simulink model "untitled"  (R2023a)
settings: Solver=VariableStepAuto  StartTime=0.0  StopTime=10.0  RelTol=1e-3
(part 1 of 2)
settings Model: Creator=green  LastModifiedBy=green

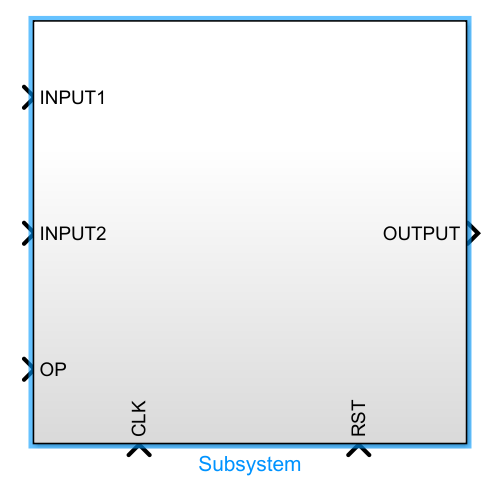
[thumbnail: Simulink's stored preview of the top-level diagram]
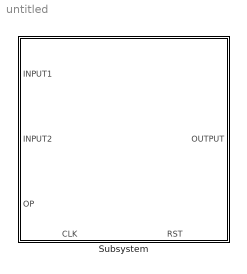
== system untitled ==
  Subsystem : Subsystem
      settings: PortSchema="{\"entries\":[{\"content\":{\"sides\":[{\"content\":{\"connectorIds\":[\"In1\",\"In2\",\"In3\"]},\"type\":\"ConnectorPlacement.EquallySpacedRectSide\",\"uuid\":\"37e95da7-9205-457f-9e39-3ce645baf6b0\"},{\"content\":{\"connectorIds\":[\"Out1\"],\"side\":\"RIGHT\"},\"type\":\"ConnectorPlacement.EquallySpacedRectSide\",\"uuid\":\"fefd857f-f6cb-479d-9e10-fdb7bd1a36ee\"},{\"content\":{\"side\":\"TOP\"},\"type\":\"ConnectorPlacement.EquallySpacedRectSide\",\"uuid\":\"cee60b90-4321-4370-ba97-5c42913d2398\"},{\"content\":{\"connectorIds\":[\"In4\",\"In5\"],\"side\":\"BOTTOM\"},\"type\":\"ConnectorPlacement.EquallySpacedRectSide\",\"uuid\":\"580bfb33-9847-4a2b-9363-58d08870a9b2\"}]},\"type\":\"ConnectorPlacement.EquallySpacedConnector\",\"uuid\":\"096c5676-b756-43ee-88e7-cfe97f701f61\"}],\"packageUris\":[\"http://schema.mathworks.com/mf0/Connector/R2020b\"],\"version\":\"1.0\"}"

== system untitled/Subsystem ==
  INPUT1 : Inport
  INPUT2 : Inport  Port=2
  OP : Inport  Port=3
  CLK : Inport  Port=4
  RST : Inport  Port=5
  AdjustingStage : Subsystem
  ComparingStage : Subsystem
  REG0 : Subsystem
      settings: PortSchema="{\"entries\":[{\"content\":{\"sides\":[{\"content\":{\"connectorIds\":[\"In1\",\"In2\",\"In3\"]},\"type\":\"ConnectorPlacement.EquallySpacedRectSide\",\"uuid\":\"0bf5a9f9-0a2e-40a8-8f36-13e781bf7f7c\"},{\"content\":{\"connectorIds\":[\"Out1\",\"Out2\",\"Out3\"],\"side\":\"RIGHT\"},\"type\":\"ConnectorPlacement.EquallySpacedRectSide\",\"uuid\":\"64de0e43-1db7-4c2b-a11f-50a8f2372dfb\"},{\"content\":{\"side\":\"TOP\"},\"type\":\"ConnectorPlacement.EquallySpacedRectSide\",\"uuid\":\"47007070-ff58-4456-a49f-5fa02446871f\"},{\"content\":{\"connectorIds\":[\"In4\",\"In5\"],\"side\":\"BOTTOM\"},\"type\":\"ConnectorPlacement.EquallySpacedRectSide\",\"uuid\":\"deeacdac-dd8e-4111-be34-c34c5f9ad249\"}]},\"type\":\"ConnectorPlacement.EquallySpacedConnector\",\"uuid\":\"bf4352da-4f56-4c40-9a35-5ffeed5d8f33\"}],\"packageUris\":[\"http://schema.mathworks.com/mf0/Connector/R2020b\"],\"version\":\"1.0\"}"
      mask Display:
      | port_label('output', 1, 'REG0_INPUT1_OUT');
      | port_label('output', 2, 'REG0_INPUT2_OUT');
      | port_label('output', 3, 'REG0_OP_OUT');
  REG1 : Subsystem
      settings: PortSchema="{\"entries\":[{\"content\":{\"sides\":[{\"content\":{\"connectorIds\":[\"In1\",\"In2\",\"In3\",\"In4\",\"In5\",\"In6\",\"In7\",\"In8\"]},\"type\":\"ConnectorPlacement.EquallySpacedRectSide\",\"uuid\":\"9e1207e4-08ad-44e3-9c00-a9750af8a307\"},{\"content\":{\"connectorIds\":[\"Out1\",\"Out2\",\"Out3\",\"Out4\",\"Out5\",\"Out6\",\"Out7\",\"Out8\"],\"side\":\"RIGHT\"},\"type\":\"ConnectorPlacement.EquallySpacedRectSide\",\"uuid\":\"02430975-5577-49fa-ae01-2c7f0237ca90\"},{\"content\":{\"side\":\"TOP\"},\"type\":\"ConnectorPlacement.EquallySpacedRectSide\",\"uuid\":\"2f56d54c-2170-4dac-9216-b09e8eed7f96\"},{\"content\":{\"connectorIds\":[\"In9\",\"In10\"],\"side\":\"BOTTOM\"},\"type\":\"ConnectorPlacement.EquallySpacedRectSide\",\"uuid\":\"f0451ad4-7d82-4ea8-9575-37119c4c4164\"}]},\"type\":\"ConnectorPlacement.EquallySpacedConnector\",\"uuid\":\"88e41896-9e94-456f-8982-875c164cfc6d\"}],\"packageUris\":[\"http://schema.mathworks.com/mf0/Connector/R2020b\"],\"version\":\"1.0\"}"
      mask Display:
      | port_label('output', 1, 'REG1_GRT_MAN_OUT');
      | port_label('output', 2, 'REG1_SML_MAN_OUT');
      | port_label('output', 3, 'REG1_GRT_EXP_OUT');
      | port_label('output', 4, 'REG1_OP_OUT');
      | port_label('output', 5, 'REG1_OFF_OUT');
      | port_label('output', 6, 'REG1_ERR_OUT');
      | port_label('output', 7, 'REG1_SIG_OUT');
      | port_label('output', 8, 'REG1_SKIP_OUT');
  Subsystem : Subsystem
      settings: PortSchema="{\"entries\":[{\"content\":{\"sides\":[{\"content\":{\"connectorIds\":[\"In1\",\"In2\",\"In3\",\"In4\",\"In5\"]},\"type\":\"ConnectorPlacement.EquallySpacedRectSide\",\"uuid\":\"271f7499-cbf5-43d7-a36f-68a92dde91c3\"},{\"content\":{\"connectorIds\":[\"Out1\",\"Out2\",\"Out3\",\"Out4\",\"Out5\"],\"side\":\"RIGHT\"},\"type\":\"ConnectorPlacement.EquallySpacedRectSide\",\"uuid\":\"c829676f-f788-46a0-9fbf-cc0d28732a72\"},{\"content\":{\"side\":\"TOP\"},\"type\":\"ConnectorPlacement.EquallySpacedRectSide\",\"uuid\":\"0b615c9c-1d4c-432e-addf-ad86eb345932\"},{\"content\":{\"connectorIds\":[\"In6\",\"In7\"],\"side\":\"BOTTOM\"},\"type\":\"ConnectorPlacement.EquallySpacedRectSide\",\"uuid\":\"741bad5f-e323-4eab-96d6-6de12d9467e0\"}]},\"type\":\"ConnectorPlacement.EquallySpacedConnector\",\"uuid\":\"c092d22a-06ee-42ed-a6ff-dc5cfd987c26\"}],\"packageUris\":[\"http://schema.mathworks.com/mf0/Connector/R2020b\"],\"version\":\"1.0\"}"
      mask Display:
      | port_label('output', 1, 'REG2_MAN_OUT');
      | port_label('output', 2, 'REG2_EXP_OUT');
      | port_label('output', 3, 'REG2_ERR_OUT');
      | port_label('output', 4, 'REG2_SIG_OUT');
      | port_label('output', 5, 'REG2_SKIP_OUT');
  Subsystem1 : Subsystem
      settings: PortSchema="{\"entries\":[{\"content\":{\"sides\":[{\"content\":{\"connectorIds\":[\"In1\"]},\"type\":\"ConnectorPlacement.EquallySpacedRectSide\",\"uuid\":\"4eea08a2-4b46-4ed3-b242-b8d68ae14b1d\"},{\"content\":{\"connectorIds\":[\"Out1\"],\"side\":\"RIGHT\"},\"type\":\"ConnectorPlacement.EquallySpacedRectSide\",\"uuid\":\"bd76014b-9e49-4f9b-8f52-6c35a06cb956\"},{\"content\":{\"side\":\"TOP\"},\"type\":\"ConnectorPlacement.EquallySpacedRectSide\",\"uuid\":\"e81f4656-2d66-443e-b83c-e94aced2d1e6\"},{\"content\":{\"connectorIds\":[\"In2\",\"In3\"],\"side\":\"BOTTOM\"},\"type\":\"ConnectorPlacement.EquallySpacedRectSide\",\"uuid\":\"afa62644-27c9-45a7-ab20-cd97c66f7d54\"}]},\"type\":\"ConnectorPlacement.EquallySpacedConnector\",\"uuid\":\"b17d71c5-ec26-422c-beb5-b1687da0b41b\"}],\"packageUris\":[\"http://schema.mathworks.com/mf0/Connector/R2020b\"],\"version\":\"1.0\"}"
      mask Display: port_label('output', 1, 'REG3_FINAL_OUT');
  SummingStage : Subsystem
  OUTPUT : Outport
  wires:
  INPUT1/1 -> REG0/1(INPUT1)
  INPUT2/1 -> REG0/2(INPUT2)
  OP/1 -> REG0/3(OP)
  REG1/1(REG1_GRT_MAN_OUT) -> SummingStage/1(GRT_MAN)
  REG1/2(REG1_SML_MAN_OUT) -> SummingStage/2(SML_MAN)
  REG1/3(REG1_GRT_EXP_OUT) -> SummingStage/3(GRT_EXP)
  REG1/4(Out4) -> SummingStage/4(OP_IN)
  REG1/5(Out6) -> SummingStage/5(OFF)
  REG1/6(REG0_INPUT2_OUT) -> SummingStage/6(ERR_IN)
  ComparingStage/1(GRT_MAN) -> REG1/1(INPUT1)
  ComparingStage/2(SML_MAN) -> REG1/2(INPUT2)
  ComparingStage/3(GRT_EXP) -> REG1/3(OP)
  ComparingStage/4(OP_OUT) -> REG1/4(In4)
  ComparingStage/5(OFF) -> REG1/5(In5)
  ComparingStage/6(ERR) -> REG1/6(In6)
  ComparingStage/7(SIG_OUT) -> REG1/7(In7)
  ComparingStage/8(SKIP) -> REG1/8(In8)
  REG0/1(REG0_INPUT1_OUT) -> ComparingStage/1(INPUT1)
  REG0/2(REG0_INPUT2_OUT) -> ComparingStage/2(INPUT2)
  REG0/3(REG0_OP_OUT) -> ComparingStage/3(OP_IN)
  Subsystem/1(SIG_IN) -> AdjustingStage/1(SIG_IN)
  Subsystem/2(EXP_IN) -> AdjustingStage/2(EXP_IN)
  Subsystem/3(MAN_IN) -> AdjustingStage/3(MAN_IN)
  Subsystem/4(SKIP) -> AdjustingStage/4(SKIP)
  Subsystem/5(ERR) -> AdjustingStage/5(ERR)
  AdjustingStage/1(FINAL) -> Subsystem1/1(FINAL)
  Subsystem1/1(OUTPUT) -> OUTPUT/1
  REG1/7(REG0_OP_OUT) -> Subsystem/4(In1)
  REG1/8(Out5) -> Subsystem/5(In5)
  SummingStage/1(EXP_OUT) -> Subsystem/1(EXP_OUT)
  SummingStage/2(MAN_OUT) -> Subsystem/2(MAN_OUT)
  SummingStage/3(ERR_OUT) -> Subsystem/3(ERR_OUT)
  CLK/1 -> Subsystem1/2(In2), Subsystem/6(In2), REG1/9(In1), REG0/4(In1)
  RST/1 -> Subsystem1/3(" "), Subsystem/7(In6), REG1/10(In9), REG0/5(In4)

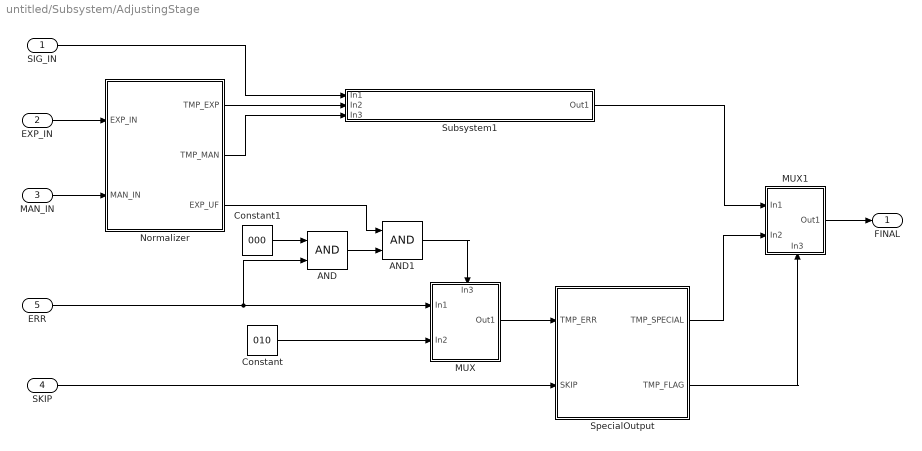
== system untitled/Subsystem/AdjustingStage ==
  SIG_IN : Inport
  EXP_IN : Inport  Port=2
  MAN_IN : Inport  Port=3
  SKIP : Inport  Port=4
  ERR : Inport  Port=5
  AND : Logic  IconShape=distinctive  AllPortsSameDT=off  OutDataTypeStr=boolean
  AND1 : Logic  IconShape=distinctive  AllPortsSameDT=off  OutDataTypeStr=boolean
  Constant : Constant  Value=010
  Constant1 : Constant  Value=000
  MUX : Subsystem
      settings: PortSchema="{\"entries\":[{\"content\":{\"sides\":[{\"content\":{\"connectorIds\":[\"In1\",\"In2\"]},\"type\":\"ConnectorPlacement.EquallySpacedRectSide\",\"uuid\":\"02237fdb-f6d2-40a5-a89d-615b1276a356\"},{\"content\":{\"connectorIds\":[\"Out1\"],\"side\":\"RIGHT\"},\"type\":\"ConnectorPlacement.EquallySpacedRectSide\",\"uuid\":\"c17ca903-72dc-4957-8b60-9b383ee3dd39\"},{\"content\":{\"connectorIds\":[\"In3\"],\"side\":\"TOP\"},\"type\":\"ConnectorPlacement.EquallySpacedRectSide\",\"uuid\":\"219c4bad-e6ed-4335-8de0-d349761dec7d\"},{\"content\":{\"side\":\"BOTTOM\"},\"type\":\"ConnectorPlacement.EquallySpacedRectSide\",\"uuid\":\"0b6946f8-6155-485f-9c00-8ea261957314\"}]},\"type\":\"ConnectorPlacement.EquallySpacedConnector\",\"uuid\":\"0d7d6bc1-a9f3-4da0-99e5-370e9c8c4307\"}],\"packageUris\":[\"http://schema.mathworks.com/mf0/Connector/R2020b\"],\"version\":\"1.0\"}"
      mask Display:
      | port_label('input', 1, '0');
      | port_label('input', 2, '1');
      | port_label('input', 3, '');
      | port_label('output', 1, 'TMP_ERR');
  MUX1 : Subsystem
      settings: PortSchema="{\"entries\":[{\"content\":{\"sides\":[{\"content\":{\"connectorIds\":[\"In1\",\"In2\"]},\"type\":\"ConnectorPlacement.EquallySpacedRectSide\",\"uuid\":\"842b9b46-49a9-41ee-9a28-1377e2337a4a\"},{\"content\":{\"connectorIds\":[\"Out1\"],\"side\":\"RIGHT\"},\"type\":\"ConnectorPlacement.EquallySpacedRectSide\",\"uuid\":\"ea0c104d-8346-410c-81be-ba3451b043ed\"},{\"content\":{\"side\":\"TOP\"},\"type\":\"ConnectorPlacement.EquallySpacedRectSide\",\"uuid\":\"b2cb6a72-8c96-408f-a410-13c771d951b5\"},{\"content\":{\"connectorIds\":[\"In3\"],\"side\":\"BOTTOM\"},\"type\":\"ConnectorPlacement.EquallySpacedRectSide\",\"uuid\":\"c054fb93-c4d9-4237-82f7-6296c0c755bf\"}]},\"type\":\"ConnectorPlacement.EquallySpacedConnector\",\"uuid\":\"8a04c4bc-3f9a-4cc9-9da7-f908a4e56a14\"}],\"packageUris\":[\"http://schema.mathworks.com/mf0/Connector/R2020b\"],\"version\":\"1.0\"}"
      mask Display:
      | port_label('input', 1, '0');
      | port_label('input', 2, '1');
      | port_label('input', 3, '');
      | port_label('output', 1, 'FINAL');
  Normalizer : Subsystem
  SpecialOutput : Subsystem
  Subsystem1 : Subsystem
      mask Display: disp('SIGN_IN & TMP_EXP & TMP_MAN(22 downto 0)');
  FINAL : Outport
  wires:
  EXP_IN/1 -> Normalizer/1(EXP_IN)
  MAN_IN/1 -> Normalizer/2(MAN_IN)
  Constant1/1 -> AND/1
  AND/1 -> AND1/2
  SIG_IN/1 -> Subsystem1/1(In1)
  ERR/1 -> MUX/1(In1), AND/2
  Normalizer/3(EXP_UF) -> AND1/1
  Normalizer/2(TMP_MAN) -> Subsystem1/3(In3)
  Normalizer/1(TMP_EXP) -> Subsystem1/2(In2)
  Subsystem1/1(Out1) -> MUX1/1(In1)
  AND1/1 -> MUX/3(In3)
  Constant/1 -> MUX/2(In2)
  MUX/1(Out1) -> SpecialOutput/1(TMP_ERR)
  SKIP/1 -> SpecialOutput/2(SKIP)
  SpecialOutput/1(TMP_SPECIAL) -> MUX1/2(In2)
  SpecialOutput/2(TMP_FLAG) -> MUX1/3(In3)
  MUX1/1(Out1) -> FINAL/1

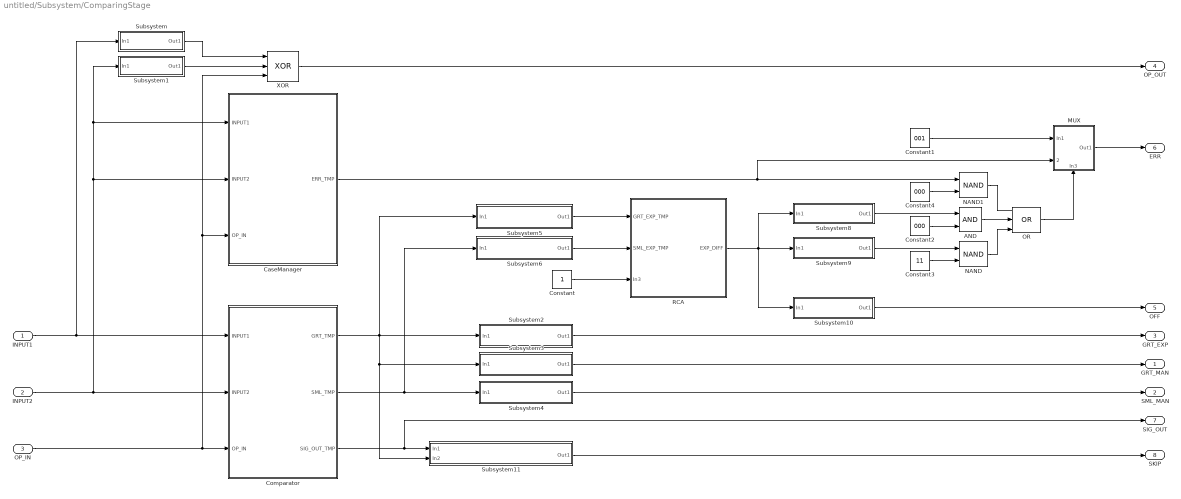
== system untitled/Subsystem/ComparingStage ==
  INPUT1 : Inport
  INPUT2 : Inport  Port=2
  OP_IN : Inport  Port=3
  AND : Logic  IconShape=distinctive  AllPortsSameDT=off  OutDataTypeStr=boolean
  CaseManager : Subsystem
  Comparator : Subsystem
  Constant : Constant
  Constant1 : Constant  Value=001
  Constant2 : Constant  Value=000
  Constant3 : Constant  Value=11
  Constant4 : Constant  Value=000
  MUX : Subsystem
      settings: PortSchema="{\"entries\":[{\"content\":{\"sides\":[{\"content\":{\"connectorIds\":[\"In1\",\"In2\"]},\"type\":\"ConnectorPlacement.EquallySpacedRectSide\",\"uuid\":\"842b9b46-49a9-41ee-9a28-1377e2337a4a\"},{\"content\":{\"connectorIds\":[\"Out1\"],\"side\":\"RIGHT\"},\"type\":\"ConnectorPlacement.EquallySpacedRectSide\",\"uuid\":\"ea0c104d-8346-410c-81be-ba3451b043ed\"},{\"content\":{\"side\":\"TOP\"},\"type\":\"ConnectorPlacement.EquallySpacedRectSide\",\"uuid\":\"b2cb6a72-8c96-408f-a410-13c771d951b5\"},{\"content\":{\"connectorIds\":[\"In3\"],\"side\":\"BOTTOM\"},\"type\":\"ConnectorPlacement.EquallySpacedRectSide\",\"uuid\":\"7dffa714-6c75-4a20-a8ae-62c0d85104c3\"}]},\"type\":\"ConnectorPlacement.EquallySpacedConnector\",\"uuid\":\"8a04c4bc-3f9a-4cc9-9da7-f908a4e56a14\"}],\"packageUris\":[\"http://schema.mathworks.com/mf0/Connector/R2020b\"],\"version\":\"1.0\"}"
      mask Display:
      | port_label('input', 1, '0');
      | port_label('input', 2, '1');
      | port_label('input', 3, '');
      | port_label('output', 1, 'ERR');
  NAND : Logic  Operator=NAND  IconShape=distinctive  AllPortsSameDT=off  OutDataTypeStr=boolean
  NAND1 : Logic  Operator=NAND  IconShape=distinctive  AllPortsSameDT=off  OutDataTypeStr=boolean
  OR : Logic  Operator=OR  Inputs=3  IconShape=distinctive  AllPortsSameDT=off  OutDataTypeStr=boolean
  RCA : Subsystem
      mask Display:
      | port_label('input', 1, 'GRT_EXP_TMP');
      | port_label('input', 2, 'SML_EXP_TMP');
      | port_label('input', 3, '');
      | port_label('output', 1, 'EXP_DIFF');
  Subsystem : Subsystem
      mask Display: disp('INPUT1(31)');
  Subsystem1 : Subsystem
      mask Display: disp('INPUT2(31)');
  Subsystem10 : Subsystem
      mask Display: disp('EXP_DIFF(4 downto 0)');
  Subsystem11 : Subsystem
      mask Display: disp('SIG_OUT_TMP & GRT_TMP(30 downto 0)');
  Subsystem2 : Subsystem
      mask Display: disp('GRT_TMP(30 downto 23)');
  Subsystem3 : Subsystem
      mask Display: disp('GRT_TMP(22 downto 0)');
  Subsystem4 : Subsystem
      mask Display: disp('SML_TMP(22 downto 0)');
  Subsystem5 : Subsystem
      mask Display: disp('GRT_TMP(30 downto 23)');
  Subsystem6 : Subsystem
      mask Display: disp('SML_TMP(30 downto 23)');
  Subsystem8 : Subsystem
      mask Display: disp('EXP_DIFF(7 downto 5)');
  Subsystem9 : Subsystem
      mask Display: disp('EXP_DIFF(4 downto 3)');
  XOR : Logic  Operator=XOR  Inputs=3  IconShape=distinctive  AllPortsSameDT=off  OutDataTypeStr=boolean
  GRT_MAN : Outport
  SML_MAN : Outport  Port=2
  GRT_EXP : Outport  Port=3
  OP_OUT : Outport  Port=4
  OFF : Outport  Port=5
  ERR : Outport  Port=6
  SIG_OUT : Outport  Port=7
  SKIP : Outport  Port=8
  wires:
  OP_IN/1 -> XOR/3, CaseManager/3(OP_IN), Comparator/3(OP_IN)
  Subsystem1/1(Out1) -> XOR/2
  Subsystem/1(Out1) -> XOR/1
  INPUT2/1 -> Subsystem1/1(In1), CaseManager/1(INPUT1), CaseManager/2(INPUT2), Comparator/2(INPUT2)
  INPUT1/1 -> Subsystem/1(In1), Comparator/1(INPUT1)
  XOR/1 -> OP_OUT/1
  Comparator/3(SIG_OUT_TMP) -> Subsystem11/1(In1), SIG_OUT/1
  Comparator/1(GRT_TMP) -> Subsystem2/1(In1), Subsystem5/1(In1), Subsystem3/1(In1), Subsystem11/2(In2)
  Comparator/2(SML_TMP) -> Subsystem4/1(In1), Subsystem6/1(In1)
  Subsystem2/1(Out1) -> GRT_EXP/1
  Subsystem3/1(Out1) -> GRT_MAN/1
  Subsystem4/1(Out1) -> SML_MAN/1
  Constant/1 -> RCA/3(In3)
  Subsystem5/1(Out1) -> RCA/1(GRT_EXP_TMP)
  Subsystem6/1(Out1) -> RCA/2(SML_EXP_TMP)
  CaseManager/1(ERR_TMP) -> NAND1/1, MUX/2(ERR_TMP)
  Constant1/1 -> MUX/1(In1)
  Subsystem8/1(Out1) -> AND/1
  Constant2/1 -> AND/2
  AND/1 -> OR/2
  Subsystem9/1(Out1) -> NAND/1
  Constant3/1 -> NAND/2
  NAND/1 -> OR/3
  RCA/1(EXP_DIFF) -> Subsystem10/1(In1), Subsystem8/1(In1), Subsystem9/1(In1)
  OR/1 -> MUX/3(In3)
  MUX/1(Out1) -> ERR/1
  Subsystem10/1(Out1) -> OFF/1
  NAND1/1 -> OR/1
  Constant4/1 -> NAND1/2
  Subsystem11/1(Out1) -> SKIP/1

== system untitled/Subsystem/REG0 ==
  INPUT1 : Inport
  Bus Element In2 : Inport  Port=2  PortName=INPUT2  Element=signal1
  OP : Inport  Port=3
  In1 : Inport  Port=4
  In4 : Inport  Port=5
  REG0_INPUT1_OUT : Outport
  REG0_INPUT2_OUT : Outport  Port=2
  REG0_OP_OUT : Outport  Port=3
  wires:
  INPUT1/1 -> REG0_INPUT1_OUT/1

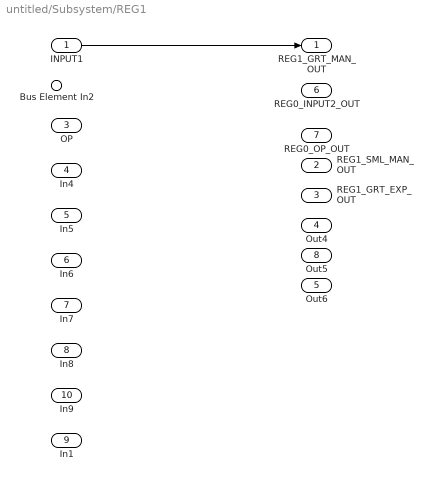
== system untitled/Subsystem/REG1 ==
  INPUT1 : Inport
  Bus Element In2 : Inport  Port=2  PortName=INPUT2  Element=signal1
  OP : Inport  Port=3
  In4 : Inport  Port=4
  In5 : Inport  Port=5
  In6 : Inport  Port=6
  In7 : Inport  Port=7
  In8 : Inport  Port=8
  In1 : Inport  Port=9
  In9 : Inport  Port=10
  REG1_GRT_MAN_OUT : Outport
  REG1_SML_MAN_OUT : Outport  Port=2
  REG1_GRT_EXP_OUT : Outport  Port=3
  Out4 : Outport  Port=4
  Out6 : Outport  Port=5
  REG0_INPUT2_OUT : Outport  Port=6
  REG0_OP_OUT : Outport  Port=7
  Out5 : Outport  Port=8
  wires:
  INPUT1/1 -> REG1_GRT_MAN_OUT/1

== system untitled/Subsystem/Subsystem ==
  EXP_OUT : Inport
  MAN_OUT : Inport  Port=2
  ERR_OUT : Inport  Port=3
  In1 : Inport  Port=4
  In5 : Inport  Port=5
  In2 : Inport  Port=6
  In6 : Inport  Port=7
  SIG_IN : Outport
  EXP_IN : Outport  Port=2
  MAN_IN : Outport  Port=3
  SKIP : Outport  Port=4
  ERR : Outport  Port=5
  wires:
  In1/1 -> ERR/1

== system untitled/Subsystem/Subsystem1 ==
  FINAL : Inport
  In2 : Inport  Port=2
  " " : Inport  Port=3
  OUTPUT : Outport
  wires:
  FINAL/1 -> OUTPUT/1

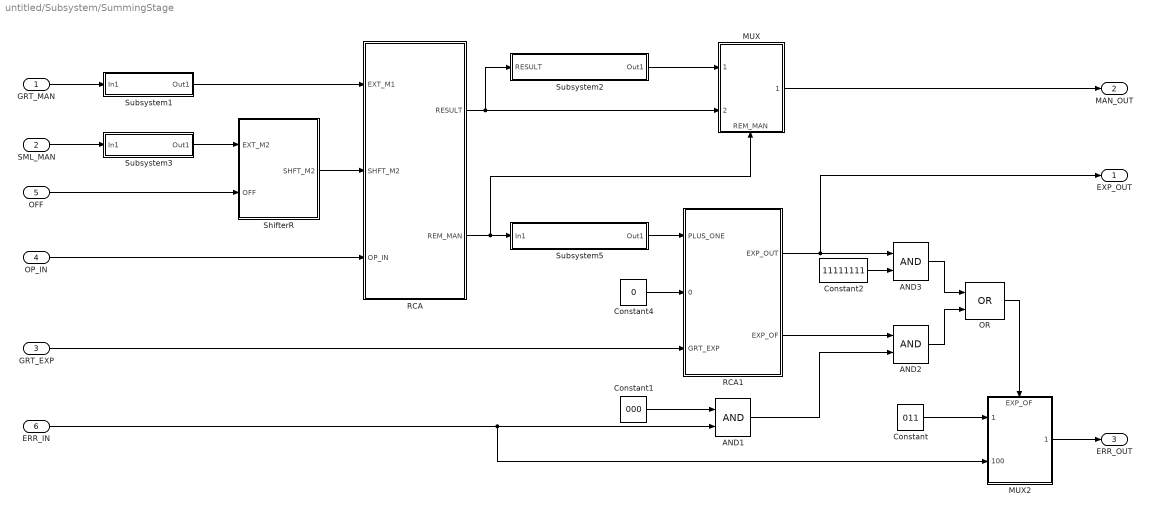
== system untitled/Subsystem/SummingStage ==
  GRT_MAN : Inport
  SML_MAN : Inport  Port=2
  GRT_EXP : Inport  Port=3
  OP_IN : Inport  Port=4
  OFF : Inport  Port=5
  ERR_IN : Inport  Port=6
  AND1 : Logic  IconShape=distinctive  AllPortsSameDT=off  OutDataTypeStr=boolean
  AND2 : Logic  IconShape=distinctive  AllPortsSameDT=off  OutDataTypeStr=boolean
  AND3 : Logic  IconShape=distinctive  AllPortsSameDT=off  OutDataTypeStr=boolean
  Constant : Constant  Value=011
  Constant1 : Constant  Value=000
  Constant2 : Constant  Value=11111111
  Constant4 : Constant  Value=0
  MUX : Subsystem
      settings: PortSchema="{\"entries\":[{\"content\":{\"sides\":[{\"content\":{\"connectorIds\":[\"In1\",\"In2\"]},\"type\":\"ConnectorPlacement.EquallySpacedRectSide\",\"uuid\":\"0af7b91d-8309-459c-bf23-687313ad86a9\"},{\"content\":{\"connectorIds\":[\"Out1\"],\"side\":\"RIGHT\"},\"type\":\"ConnectorPlacement.EquallySpacedRectSide\",\"uuid\":\"b0f577e7-d51c-44b3-9d21-1170ec3c3cca\"},{\"content\":{\"side\":\"TOP\"},\"type\":\"ConnectorPlacement.EquallySpacedRectSide\",\"uuid\":\"bf652de7-499a-4aec-b9dc-c8c3b0e92a1f\"},{\"content\":{\"connectorIds\":[\"In3\"],\"side\":\"BOTTOM\"},\"type\":\"ConnectorPlacement.EquallySpacedRectSide\",\"uuid\":\"42be33d3-65fe-49e3-b5e3-6722911f86a3\"}]},\"type\":\"ConnectorPlacement.EquallySpacedConnector\",\"uuid\":\"dd0652a8-1a35-4b5d-b245-d8ad4c57bca9\"}],\"packageUris\":[\"http://schema.mathworks.com/mf0/Connector/R2020b\"],\"version\":\"1.0\"}"
      mask Display:
      | port_label('input', 1, '0');
      | port_label('input', 2, '1');
      | port_label('input', 3, '');
      | port_label('output', 1, 'MAN_OUT');
  MUX2 : Subsystem
      settings: PortSchema="{\"entries\":[{\"content\":{\"sides\":[{\"content\":{\"connectorIds\":[\"In1\",\"In2\"]},\"type\":\"ConnectorPlacement.EquallySpacedRectSide\",\"uuid\":\"2897c680-cb6d-4652-8a24-e5e3fe3847b3\"},{\"content\":{\"connectorIds\":[\"Out1\"],\"side\":\"RIGHT\"},\"type\":\"ConnectorPlacement.EquallySpacedRectSide\",\"uuid\":\"925507d1-f46c-40a4-8c3f-56ba5c75f8db\"},{\"content\":{\"connectorIds\":[\"In3\"],\"side\":\"TOP\"},\"type\":\"ConnectorPlacement.EquallySpacedRectSide\",\"uuid\":\"081d1833-6c08-467a-9b9b-595c2258fc5e\"}]},\"type\":\"ConnectorPlacement.EquallySpacedConnector\",\"uuid\":\"f3084cfd-fad9-4a47-8091-6b741db0f626\"}],\"packageUris\":[\"http://schema.mathworks.com/mf0/Connector/R2020b\"],\"version\":\"1.0\"}"
      mask Display:
      | port_label('input', 1, '1');
      | port_label('input', 2, '0');
      | port_label('input', 3, '');
      | port_label('output', 1, 'ERR_OUT');
  OR : Logic  Operator=OR  IconShape=distinctive  AllPortsSameDT=off  OutDataTypeStr=boolean
  RCA : Subsystem
  RCA1 : Subsystem
  ShifterR : Subsystem
  Subsystem1 : Subsystem
      mask Display: disp("'1' & GRT_MAN");
  Subsystem2 : Subsystem
      mask Display: disp("'1' & RESULT(23 downto 1)");
  Subsystem3 : Subsystem
      mask Display: disp("'1' & SML_MAN");
  Subsystem5 : Subsystem
      mask Display: disp('"0000000" & REM_MAN');
  EXP_OUT : Outport
  MAN_OUT : Outport  Port=2
  ERR_OUT : Outport  Port=3
  wires:
  GRT_MAN/1 -> Subsystem1/1(In1)
  Subsystem1/1(Out1) -> RCA/1(EXT_M1)
  SML_MAN/1 -> Subsystem3/1(In1)
  OFF/1 -> ShifterR/2(OFF)
  Subsystem3/1(Out1) -> ShifterR/1(EXT_M2)
  ShifterR/1(SHFT_M2) -> RCA/2(SHFT_M2)
  OP_IN/1 -> RCA/3(OP_IN)
  RCA/1(RESULT) -> MUX/2(RESULT), Subsystem2/1(RESULT)
  Subsystem2/1(Out1) -> MUX/1('1' & RESULT(23 downto 1))
  RCA/2(REM_MAN) -> Subsystem5/1(In1), MUX/3(REM_MAN)
  Constant4/1 -> RCA1/2(0)
  GRT_EXP/1 -> RCA1/3(GRT_EXP)
  MUX2/1(ERR_OUT) -> ERR_OUT/1
  RCA1/2(EXP_OF) -> AND2/1
  RCA1/1(EXP_OUT) -> AND3/1, EXP_OUT/1
  MUX/1(MAN_OUT) -> MAN_OUT/1
  Subsystem5/1(Out1) -> RCA1/1(PLUS_ONE)
  AND1/1 -> AND2/2
  AND2/1 -> OR/2
  ERR_IN/1 -> MUX2/2(100), AND1/2
  Constant1/1 -> AND1/1
  Constant2/1 -> AND3/2
  AND3/1 -> OR/1
  OR/1 -> MUX2/3(EXP_OF)
  Constant/1 -> MUX2/1(ERR_IN)

== system untitled/Subsystem/AdjustingStage/MUX ==
  In1 : Inport
  In2 : Inport  Port=2
  In3 : Inport  Port=3
  Out1 : Outport
  wires:
  In1/1 -> Out1/1

== system untitled/Subsystem/AdjustingStage/MUX1 ==
  In1 : Inport
  In2 : Inport  Port=2
  In3 : Inport  Port=3
  Out1 : Outport
  wires:
  In1/1 -> Out1/1

== system untitled/Subsystem/AdjustingStage/Normalizer ==
  EXP_IN : Inport
  MAN_IN : Inport  Port=2
  Constant : Constant
  EightBitComparator : Subsystem
  RCA : Subsystem
      mask Display:
      | port_label('input', 1, 'SUB_EXP');
      | port_label('input', 2, 'EXP_IN');
      | port_label('input', 3, '');
      | port_label('output', 1, 'EXP_OUT');
  ReversePriorityEncoder : Subsystem
  ShifterL : Subsystem
  Subsystem : Subsystem
      mask Display: disp('"000" & MAN_OFF');
  TMP_EXP : Outport
  TMP_MAN : Outport  Port=2
  EXP_UF : Outport  Port=3
  wires:
  EXP_IN/1 -> EightBitComparator/2(EXP_IN), RCA/2(EXP_IN)
  MAN_IN/1 -> ShifterL/1(MAN_IN), ReversePriorityEncoder/1(MAN_IN)
  EightBitComparator/1(EXP_UF) -> EXP_UF/1
  ReversePriorityEncoder/1(MAN_OFF) -> Subsystem/1(In1), ShifterL/2(MAN_OFF)
  Constant/1 -> RCA/3(In3)
  ShifterL/1(MAN_OUT) -> TMP_MAN/1
  Subsystem/1(Out1) -> EightBitComparator/1(SUB_EXP), RCA/1(SUB_EXP)
  RCA/1(TMP_EXP) -> TMP_EXP/1

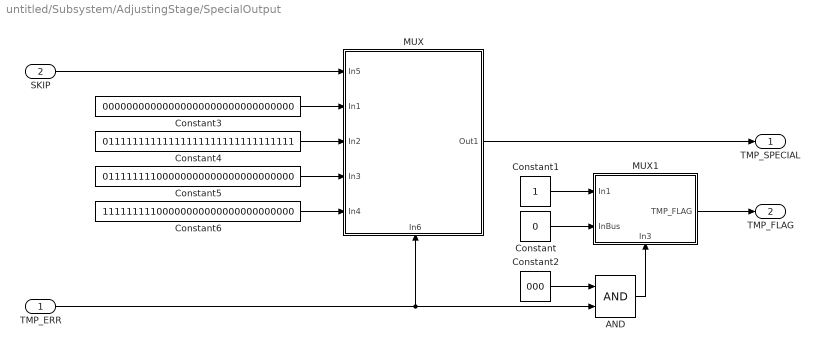
== system untitled/Subsystem/AdjustingStage/SpecialOutput ==
  TMP_ERR : Inport
  SKIP : Inport  Port=2
  AND : Logic  IconShape=distinctive  AllPortsSameDT=off  OutDataTypeStr=boolean
  Constant : Constant  Value=0
  Constant1 : Constant
  Constant2 : Constant  Value=000
  Constant3 : Constant  Value=00000000000000000000000000000000
  Constant4 : Constant  Value=01111111111111111111111111111111
  Constant5 : Constant  Value=01111111100000000000000000000000
  Constant6 : Constant  Value=11111111100000000000000000000000
  MUX : Subsystem
      settings: PortSchema="{\"entries\":[{\"content\":{\"sides\":[{\"content\":{\"connectorIds\":[\"In1\",\"In2\",\"In3\",\"In4\",\"In5\"]},\"type\":\"ConnectorPlacement.EquallySpacedRectSide\",\"uuid\":\"5e07290b-d201-45e5-8fb6-3b7645cad16a\"},{\"content\":{\"connectorIds\":[\"Out1\"],\"side\":\"RIGHT\"},\"type\":\"ConnectorPlacement.EquallySpacedRectSide\",\"uuid\":\"121e94c0-2fd9-44dd-885d-4892fcc0330c\"},{\"content\":{\"side\":\"TOP\"},\"type\":\"ConnectorPlacement.EquallySpacedRectSide\",\"uuid\":\"23c8d311-baf5-4fed-9fc8-141dbfd7a4f6\"},{\"content\":{\"connectorIds\":[\"In6\"],\"side\":\"BOTTOM\"},\"type\":\"ConnectorPlacement.EquallySpacedRectSide\",\"uuid\":\"04edf9c0-43a5-40ca-8b60-53a19ef882ba\"}]},\"type\":\"ConnectorPlacement.EquallySpacedConnector\",\"uuid\":\"00259f8c-48ac-41f9-862c-c099ddde5e22\"}],\"packageUris\":[\"http://schema.mathworks.com/mf0/Connector/R2020b\"],\"version\":\"1.0\"}"
      mask Display:
      | port_label('input', 1, '001');
      | port_label('input', 2, '010');
      | port_label('input', 3, '011');
      | port_label('input', 4, '100');
      | port_label('input', 5, '101');
      | port_label('input', 6, '');
      | port_label('output', 1, 'SPECIAL_OUTPUT');
  MUX1 : Subsystem
      settings: PortSchema="{\"entries\":[{\"content\":{\"sides\":[{\"content\":{\"connectorIds\":[\"In1\",\"In2\"]},\"type\":\"ConnectorPlacement.EquallySpacedRectSide\",\"uuid\":\"955e3f4d-4793-4010-a428-51868f7d2ec6\"},{\"content\":{\"connectorIds\":[\"Out1\"],\"side\":\"RIGHT\"},\"type\":\"ConnectorPlacement.EquallySpacedRectSide\",\"uuid\":\"61b0983f-db62-4cba-b7ea-2cfa5c22181b\"},{\"content\":{\"side\":\"TOP\"},\"type\":\"ConnectorPlacement.EquallySpacedRectSide\",\"uuid\":\"cc39428d-c27c-44a8-827d-5c2b33ddbbc2\"},{\"content\":{\"connectorIds\":[\"In3\"],\"side\":\"BOTTOM\"},\"type\":\"ConnectorPlacement.EquallySpacedRectSide\",\"uuid\":\"33e3dd30-1127-4c87-9803-948a15f9baaf\"}]},\"type\":\"ConnectorPlacement.EquallySpacedConnector\",\"uuid\":\"928a7d94-0050-4942-8dd5-27d2345332b8\"}],\"packageUris\":[\"http://schema.mathworks.com/mf0/Connector/R2020b\"],\"version\":\"1.0\"}"
      mask Display:
      | port_label('input', 1, '0');
      | port_label('input', 2, '1');
      | port_label('input', 3, '');
      | port_label('output', 1, 'SPECIAL_FLAG');
  TMP_SPECIAL : Outport
  TMP_FLAG : Outport  Port=2
  wires:
  TMP_ERR/1 -> AND/2, MUX/6(In6)
  MUX/1(Out1) -> TMP_SPECIAL/1
  SKIP/1 -> MUX/1(In5)
  Constant2/1 -> AND/1
  Constant1/1 -> MUX1/1(In1)
  Constant/1 -> MUX1/2(InBus)
  AND/1 -> MUX1/3(In3)
  MUX1/1(TMP_FLAG) -> TMP_FLAG/1
  Constant3/1 -> MUX/2(In1)
  Constant4/1 -> MUX/3(In2)
  Constant5/1 -> MUX/4(In3)
  Constant6/1 -> MUX/5(In4)

== system untitled/Subsystem/AdjustingStage/Subsystem1 ==
  In1 : Inport
  In2 : Inport  Port=2
  In3 : Inport  Port=3
  Out1 : Outport
  wires:
  In1/1 -> Out1/1

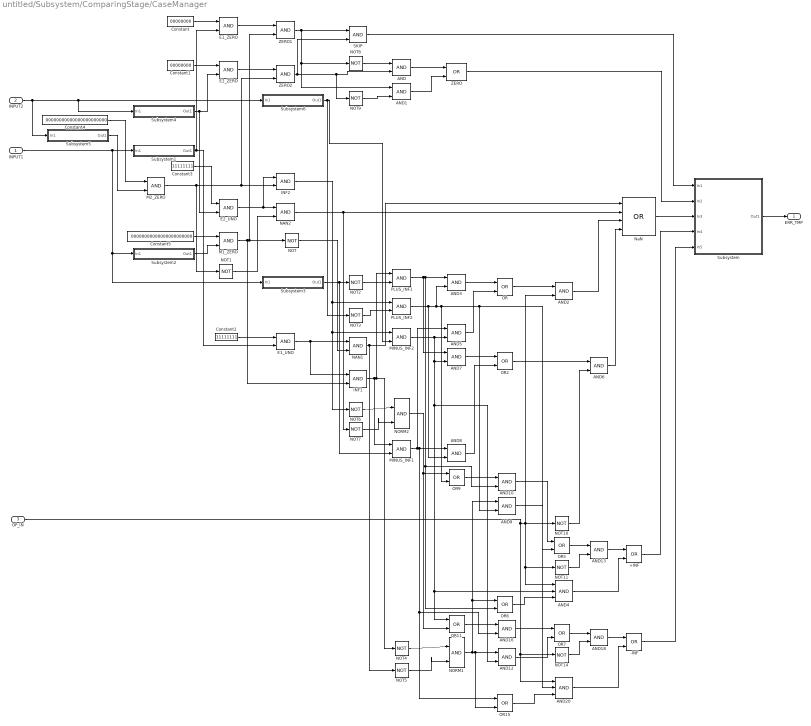
== system untitled/Subsystem/ComparingStage/CaseManager ==
  INPUT1 : Inport
  INPUT2 : Inport  Port=2
  OP_IN : Inport  Port=3
  +INF : Logic  Operator=OR  IconShape=distinctive  AllPortsSameDT=off  OutDataTypeStr=boolean
  -INF : Logic  Operator=OR  IconShape=distinctive  AllPortsSameDT=off  OutDataTypeStr=boolean
  AND{,1..3,5..10,12..13,16,18} (14 alike) : Logic  IconShape=distinctive  AllPortsSameDT=off  OutDataTypeStr=boolean
  AND20 : Logic  Inputs=3  IconShape=distinctive  AllPortsSameDT=off  OutDataTypeStr=boolean
  AND4 : Logic  Inputs=3  IconShape=distinctive  AllPortsSameDT=off  OutDataTypeStr=boolean
  Constant : Constant  Value=00000000
  Constant1 : Constant  Value=00000000
  Constant2 : Constant  Value=11111111
  Constant3 : Constant  Value=11111111
  Constant4 : Constant  Value=00000000000000000000000
  Constant5 : Constant  Value=00000000000000000000000
  E1_UNO : Logic  IconShape=distinctive  AllPortsSameDT=off  OutDataTypeStr=boolean
  E1_ZERO : Logic  IconShape=distinctive  AllPortsSameDT=off  OutDataTypeStr=boolean
  E2_UNO : Logic  IconShape=distinctive  AllPortsSameDT=off  OutDataTypeStr=boolean
  E2_ZERO : Logic  IconShape=distinctive  AllPortsSameDT=off  OutDataTypeStr=boolean
  INF1 : Logic  IconShape=distinctive  AllPortsSameDT=off  OutDataTypeStr=boolean
  INF2 : Logic  IconShape=distinctive  AllPortsSameDT=off  OutDataTypeStr=boolean
  M1_ZERO : Logic  IconShape=distinctive  AllPortsSameDT=off  OutDataTypeStr=boolean
  M2_ZERO : Logic  IconShape=distinctive  AllPortsSameDT=off  OutDataTypeStr=boolean
  MINUS_INF1 : Logic  IconShape=distinctive  AllPortsSameDT=off  OutDataTypeStr=boolean
  MINUS_INF2 : Logic  IconShape=distinctive  AllPortsSameDT=off  OutDataTypeStr=boolean
  NAN1 : Logic  IconShape=distinctive  AllPortsSameDT=off  OutDataTypeStr=boolean
  NAN2 : Logic  IconShape=distinctive  AllPortsSameDT=off  OutDataTypeStr=boolean
  NORM1 : Logic  IconShape=distinctive  AllPortsSameDT=off  OutDataTypeStr=boolean
  NORM2 : Logic  IconShape=distinctive  AllPortsSameDT=off  OutDataTypeStr=boolean
  NOT{,1..11,14} (13 alike) : Logic  Operator=NOT  IconShape=distinctive  AllPortsSameDT=off  OutDataTypeStr=boolean
  NaN : Logic  Operator=OR  Inputs=4  IconShape=distinctive  AllPortsSameDT=off  OutDataTypeStr=boolean
  OR{,2,5..7,9,11,15} (8 alike) : Logic  Operator=OR  IconShape=distinctive  AllPortsSameDT=off  OutDataTypeStr=boolean
  PLUS_INF1 : Logic  IconShape=distinctive  AllPortsSameDT=off  OutDataTypeStr=boolean
  PLUS_INF2 : Logic  IconShape=distinctive  AllPortsSameDT=off  OutDataTypeStr=boolean
  SKIP : Logic  IconShape=distinctive  AllPortsSameDT=off  OutDataTypeStr=boolean
  Subsystem : Subsystem
      mask Display:
      | port_label('input', 1, '001');
      | port_label('input', 2, '010');
      | port_label('input', 3, '011');
      | port_label('input', 4, '100');
      | port_label('input', 5, '101');
      | port_label('output', 1, 'xy');
  Subsystem1 : Subsystem
      mask Display: disp('INPUT1(30 downto 23)');
  Subsystem2 : Subsystem
      mask Display: disp('INPUT1(22 downto 0)');
  Subsystem3 : Subsystem
      mask Display: disp('INPUT1(31)');
  Subsystem4 : Subsystem
      mask Display: disp('INPUT2(30 downto 23)');
  Subsystem5 : Subsystem
      mask Display: disp('INPUT2(22 downto 0)');
  Subsystem6 : Subsystem
      mask Display: disp('INPUT2(31)');
  ZERO : Logic  Operator=OR  IconShape=distinctive  AllPortsSameDT=off  OutDataTypeStr=boolean
  ZERO1 : Logic  IconShape=distinctive  AllPortsSameDT=off  OutDataTypeStr=boolean
  ZERO2 : Logic  IconShape=distinctive  AllPortsSameDT=off  OutDataTypeStr=boolean
  ERR_TMP : Outport
  wires:
  M1_ZERO/1 -> ZERO1/2, NOT/1, INF1/2
  INPUT2/1 -> Subsystem6/1(In1), Subsystem4/1(In1), Subsystem5/1(In1)
  Subsystem4/1(Out1) -> E2_ZERO/2, E2_UNO/2
  OR11/1 -> AND16/1
  INF1/1 -> NOT4/1, PLUS_INF1/1, MINUS_INF1/1
  Constant1/1 -> E2_ZERO/1
  AND16/1 -> OR7/1
  ZERO2/1 -> AND/2, NOT9/1, SKIP/2
  Constant4/1 -> M2_ZERO/1
  OR5/1 -> AND13/1
  NOT10/1 -> AND6/2
  Subsystem5/1(Out1) -> M2_ZERO/2
  INPUT1/1 -> Subsystem3/1(In1), Subsystem2/1(In1), Subsystem1/1(In1)
  Constant/1 -> E1_ZERO/1
  Subsystem1/1(Out1) -> E1_UNO/2, E1_ZERO/2
  Constant3/1 -> E2_UNO/1
  M2_ZERO/1 -> INF2/2, ZERO2/2, NOT1/1
  OR6/1 -> AND4/3
  Subsystem6/1(Out1) -> MINUS_INF2/2, NOT3/1
  Constant5/1 -> M1_ZERO/1
  AND7/1 -> OR2/1
  OR2/1 -> AND6/1
  Subsystem2/1(Out1) -> M1_ZERO/2
  AND10/1 -> OR5/1
  E1_ZERO/1 -> ZERO1/1
  E2_ZERO/1 -> ZERO2/1
  E2_UNO/1 -> NAN2/1, INF2/1
  NOT1/1 -> NAN2/2
  Subsystem3/1(Out1) -> MINUS_INF1/2, NOT2/1
  Constant2/1 -> E1_UNO/1
  ZERO1/1 -> NOT8/1, AND1/1, SKIP/1
  INF2/1 -> MINUS_INF2/1, NOT6/1, PLUS_INF2/1
  NAN2/1 -> NaN/2, NOT7/1
  NOT/1 -> NAN1/2
  AND9/1 -> OR5/2
  E1_UNO/1 -> NAN1/1, INF1/1
  SKIP/1 -> Subsystem/1(In1)
  OR/1 -> AND2/1
  NOT8/1 -> AND/1
  ZERO/1 -> Subsystem/2(In2)
  NOT9/1 -> AND1/2
  NOT2/1 -> PLUS_INF1/2
  NOT3/1 -> PLUS_INF2/2
  NAN1/1 -> NOT5/1, NaN/1
  NOT6/1 -> NORM2/1
  MINUS_INF2/1 -> AND4/2, OR11/1, AND12/2, AND7/2, AND5/2
  AND2/1 -> NaN/3
  OR15/1 -> AND20/3
  NOT7/1 -> NORM2/2
  AND/1 -> ZERO/1
  AND1/1 -> ZERO/2
  PLUS_INF1/1 -> AND10/2, OR6/2, AND3/1, AND7/1
  PLUS_INF2/1 -> AND20/2, AND9/2, OR9/2, AND3/2, AND8/2
  NORM2/1 -> OR9/1, OR11/2
  OR9/1 -> AND10/1
  MINUS_INF1/1 -> AND16/2, OR15/1, AND8/1, AND5/1
  OP_IN/1 -> NOT14/1, AND20/1, NOT11/1, AND4/1, AND2/2, NOT10/1
  NOT4/1 -> NORM1/1
  AND13/1 -> +INF/1
  NOT5/1 -> NORM1/2
  AND5/1 -> OR/2
  AND3/1 -> OR/1
  AND8/1 -> OR2/2
  NORM1/1 -> AND12/1, OR15/2, OR6/1, AND9/1
  AND12/1 -> OR7/2
  NOT11/1 -> AND13/2
  AND4/1 -> +INF/2
  OR7/1 -> AND18/1
  NOT14/1 -> AND18/2
  AND20/1 -> -INF/2
  AND6/1 -> NaN/4
  AND18/1 -> -INF/1
  NaN/1 -> Subsystem/3(In3)
  +INF/1 -> Subsystem/4(In4)
  -INF/1 -> Subsystem/5(In5)
  Subsystem/1(Out1) -> ERR_TMP/1

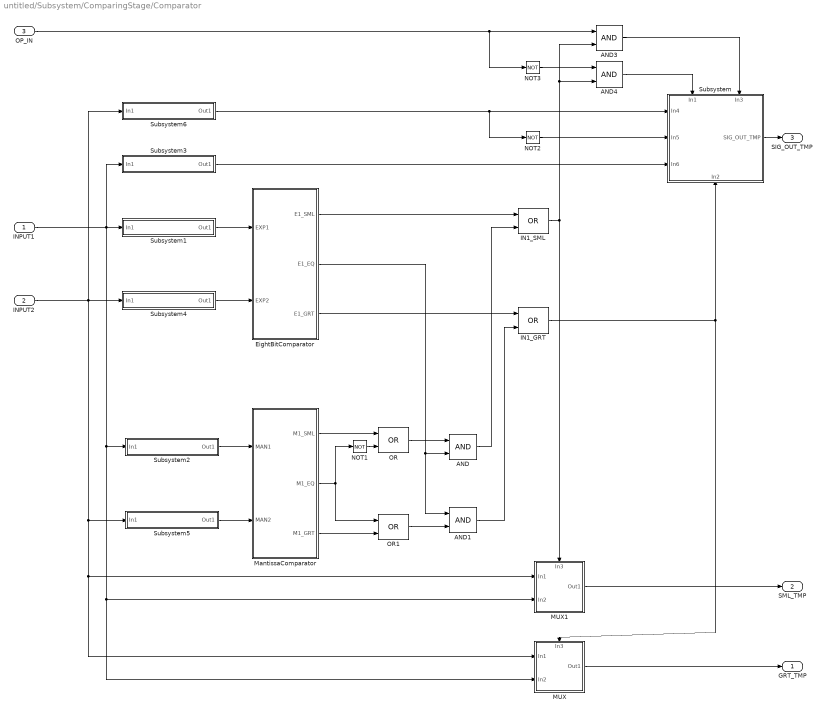
== system untitled/Subsystem/ComparingStage/Comparator ==
  INPUT1 : Inport
  INPUT2 : Inport  Port=2
  OP_IN : Inport  Port=3
  AND{,1,3..4} (4 alike) : Logic  IconShape=distinctive  AllPortsSameDT=off  OutDataTypeStr=boolean
  EightBitComparator : Subsystem
  IN1_GRT : Logic  Operator=OR  IconShape=distinctive  AllPortsSameDT=off  OutDataTypeStr=boolean
  IN1_SML : Logic  Operator=OR  IconShape=distinctive  AllPortsSameDT=off  OutDataTypeStr=boolean
  MUX : Subsystem
      settings: PortSchema="{\"entries\":[{\"content\":{\"sides\":[{\"content\":{\"connectorIds\":[\"In1\",\"In2\"]},\"type\":\"ConnectorPlacement.EquallySpacedRectSide\",\"uuid\":\"955e3f4d-4793-4010-a428-51868f7d2ec6\"},{\"content\":{\"connectorIds\":[\"Out1\"],\"side\":\"RIGHT\"},\"type\":\"ConnectorPlacement.EquallySpacedRectSide\",\"uuid\":\"61b0983f-db62-4cba-b7ea-2cfa5c22181b\"},{\"content\":{\"connectorIds\":[\"In3\"],\"side\":\"TOP\"},\"type\":\"ConnectorPlacement.EquallySpacedRectSide\",\"uuid\":\"cc39428d-c27c-44a8-827d-5c2b33ddbbc2\"},{\"content\":{\"side\":\"BOTTOM\"},\"type\":\"ConnectorPlacement.EquallySpacedRectSide\",\"uuid\":\"9971c126-fda8-43cf-95f1-996d1a10f757\"}]},\"type\":\"ConnectorPlacement.EquallySpacedConnector\",\"uuid\":\"928a7d94-0050-4942-8dd5-27d2345332b8\"}],\"packageUris\":[\"http://schema.mathworks.com/mf0/Connector/R2020b\"],\"version\":\"1.0\"}"
      mask Display:
      | port_label('input', 1, '0');
      | port_label('input', 2, '1');
      | port_label('input', 3, '');
      | port_label('output', 1, 'GRT_IN');
  MUX1 : Subsystem
      settings: PortSchema="{\"entries\":[{\"content\":{\"sides\":[{\"content\":{\"connectorIds\":[\"In1\",\"In2\"]},\"type\":\"ConnectorPlacement.EquallySpacedRectSide\",\"uuid\":\"955e3f4d-4793-4010-a428-51868f7d2ec6\"},{\"content\":{\"connectorIds\":[\"Out1\"],\"side\":\"RIGHT\"},\"type\":\"ConnectorPlacement.EquallySpacedRectSide\",\"uuid\":\"61b0983f-db62-4cba-b7ea-2cfa5c22181b\"},{\"content\":{\"connectorIds\":[\"In3\"],\"side\":\"TOP\"},\"type\":\"ConnectorPlacement.EquallySpacedRectSide\",\"uuid\":\"cc39428d-c27c-44a8-827d-5c2b33ddbbc2\"},{\"content\":{\"side\":\"BOTTOM\"},\"type\":\"ConnectorPlacement.EquallySpacedRectSide\",\"uuid\":\"9971c126-fda8-43cf-95f1-996d1a10f757\"}]},\"type\":\"ConnectorPlacement.EquallySpacedConnector\",\"uuid\":\"928a7d94-0050-4942-8dd5-27d2345332b8\"}],\"packageUris\":[\"http://schema.mathworks.com/mf0/Connector/R2020b\"],\"version\":\"1.0\"}"
      mask Display:
      | port_label('input', 1, '0');
      | port_label('input', 2, '1');
      | port_label('input', 3, '');
      | port_label('output', 1, 'SML_IN');
  MantissaComparator : Subsystem
  NOT1 : Logic  Operator=NOT  IconShape=distinctive  AllPortsSameDT=off  OutDataTypeStr=boolean
  NOT2 : Logic  Operator=NOT  IconShape=distinctive  AllPortsSameDT=off  OutDataTypeStr=boolean
  NOT3 : Logic  Operator=NOT  IconShape=distinctive  AllPortsSameDT=off  OutDataTypeStr=boolean
  OR : Logic  Operator=OR  IconShape=distinctive  AllPortsSameDT=off  OutDataTypeStr=boolean
  OR1 : Logic  Operator=OR  IconShape=distinctive  AllPortsSameDT=off  OutDataTypeStr=boolean
  Subsystem : Subsystem
      settings: PortSchema="{\"entries\":[{\"content\":{\"sides\":[{\"content\":{\"connectorIds\":[\"In1\",\"In2\",\"In3\"]},\"type\":\"ConnectorPlacement.EquallySpacedRectSide\",\"uuid\":\"85ed978f-a5ad-4314-8e65-e742cb16c3e0\"},{\"content\":{\"connectorIds\":[\"Out1\"],\"side\":\"RIGHT\"},\"type\":\"ConnectorPlacement.EquallySpacedRectSide\",\"uuid\":\"ee3c3111-56fd-4f4f-af60-c880fb7254e6\"},{\"content\":{\"connectorIds\":[\"In4\",\"In5\"],\"side\":\"TOP\"},\"type\":\"ConnectorPlacement.EquallySpacedRectSide\",\"uuid\":\"21ffd9f0-f5c2-46f9-9bc9-42c69333614c\"},{\"content\":{\"connectorIds\":[\"In6\"],\"side\":\"BOTTOM\"},\"type\":\"ConnectorPlacement.EquallySpacedRectSide\",\"uuid\":\"14d88078-416f-4820-84fb-de565a5bfa6a\"}]},\"type\":\"ConnectorPlacement.EquallySpacedConnector\",\"uuid\":\"f02ada6e-bcd2-4387-83c2-32f086e4b5fe\"}],\"packageUris\":[\"http://schema.mathworks.com/mf0/Connector/R2020b\"],\"version\":\"1.0\"}"
      mask Display:
      | port_label('input', 1, 'SIG2');
      | port_label('input', 2, 'not SIG2');
      | port_label('input', 3, 'SIG1');
      | port_label('output', 1, 'OUT_SIG');
  Subsystem1 : Subsystem
      mask Display: disp('INPUT1(30 downto 23)');
  Subsystem2 : Subsystem
      mask Display: disp('INPUT1(22 downto 0)');
  Subsystem3 : Subsystem
      mask Display: disp('INPUT1(31)');
  Subsystem4 : Subsystem
      mask Display: disp('INPUT2(30 downto 23)');
  Subsystem5 : Subsystem
      mask Display: disp('INPUT2(22 downto 0)');
  Subsystem6 : Subsystem
      mask Display: disp('INPUT2(31)');
  GRT_TMP : Outport
  SML_TMP : Outport  Port=2
  SIG_OUT_TMP : Outport  Port=3
  wires:
  INPUT1/1 -> Subsystem1/1(In1), Subsystem3/1(In1), Subsystem2/1(In1), MUX/2(In2), MUX1/2(In2)
  INPUT2/1 -> Subsystem4/1(In1), Subsystem6/1(In1), Subsystem5/1(In1), MUX/1(In1), MUX1/1(In1)
  Subsystem1/1(Out1) -> EightBitComparator/1(EXP1)
  Subsystem4/1(Out1) -> EightBitComparator/2(EXP2)
  Subsystem2/1(Out1) -> MantissaComparator/1(MAN1)
  Subsystem5/1(Out1) -> MantissaComparator/2(MAN2)
  NOT1/1 -> OR/2
  MantissaComparator/2(M1_EQ) -> NOT1/1, OR1/1
  EightBitComparator/2(E1_EQ) -> AND/2, AND1/1
  OR/1 -> AND/1
  OR1/1 -> AND1/2
  MantissaComparator/1(M1_SML) -> OR/1
  MantissaComparator/3(M1_GRT) -> OR1/2
  EightBitComparator/3(E1_GRT) -> IN1_GRT/1
  AND/1 -> IN1_SML/2
  EightBitComparator/1(E1_SML) -> IN1_SML/1
  IN1_GRT/1 -> Subsystem/6(In2), MUX/3(In3)
  IN1_SML/1 -> MUX1/3(In3), AND3/2, AND4/2
  MUX/1(Out1) -> GRT_TMP/1
  MUX1/1(Out1) -> SML_TMP/1
  AND1/1 -> IN1_GRT/2
  OP_IN/1 -> AND3/1, NOT3/1
  Subsystem3/1(Out1) -> Subsystem/3(In6)
  AND3/1 -> Subsystem/5(In3)
  Subsystem6/1(Out1) -> Subsystem/1(In4), NOT2/1
  NOT2/1 -> Subsystem/2(In5)
  Subsystem/1(SIG_OUT_TMP) -> SIG_OUT_TMP/1
  NOT3/1 -> AND4/1
  AND4/1 -> Subsystem/4(In1)

== system untitled/Subsystem/ComparingStage/MUX ==
  In1 : Inport
  ERR_TMP : Inport  Port=2
  In3 : Inport  Port=3
  Out1 : Outport
  wires:
  In1/1 -> Out1/1

== system untitled/Subsystem/ComparingStage/RCA ==
  GRT_EXP_TMP : Inport
  SML_EXP_TMP : Inport  Port=2
  In3 : Inport  Port=3
  EXP_DIFF : Outport
  wires:
  GRT_EXP_TMP/1 -> EXP_DIFF/1

== system untitled/Subsystem/ComparingStage/Subsystem ==
  In1 : Inport
  Out1 : Outport
  wires:
  In1/1 -> Out1/1

== system untitled/Subsystem/ComparingStage/Subsystem1 ==
  In1 : Inport
  Out1 : Outport
  wires:
  In1/1 -> Out1/1

== system untitled/Subsystem/ComparingStage/Subsystem10 ==
  In1 : Inport
  Out1 : Outport
  wires:
  In1/1 -> Out1/1

== system untitled/Subsystem/ComparingStage/Subsystem11 ==
  In1 : Inport
  In2 : Inport  Port=2
  Out1 : Outport
  wires:
  In1/1 -> Out1/1

== system untitled/Subsystem/ComparingStage/Subsystem2 ==
  In1 : Inport
  Out1 : Outport
  wires:
  In1/1 -> Out1/1

== system untitled/Subsystem/ComparingStage/Subsystem3 ==
  In1 : Inport
  Out1 : Outport
  wires:
  In1/1 -> Out1/1

== system untitled/Subsystem/ComparingStage/Subsystem4 ==
  In1 : Inport
  Out1 : Outport
  wires:
  In1/1 -> Out1/1

== system untitled/Subsystem/ComparingStage/Subsystem5 ==
  In1 : Inport
  Out1 : Outport
  wires:
  In1/1 -> Out1/1

== system untitled/Subsystem/ComparingStage/Subsystem6 ==
  In1 : Inport
  Out1 : Outport
  wires:
  In1/1 -> Out1/1

== system untitled/Subsystem/ComparingStage/Subsystem8 ==
  In1 : Inport
  Out1 : Outport
  wires:
  In1/1 -> Out1/1

== system untitled/Subsystem/ComparingStage/Subsystem9 ==
  In1 : Inport
  Out1 : Outport
  wires:
  In1/1 -> Out1/1

== system untitled/Subsystem/SummingStage/MUX ==
  '1' & RESULT(23 downto 1) : Inport
  RESULT : Inport  Port=2
  REM_MAN : Inport  Port=3
  MAN_OUT : Outport
  wires:
  RESULT/1 -> MAN_OUT/1

== system untitled/Subsystem/SummingStage/MUX2 ==
  ERR_IN : Inport
  100 : Inport  Port=2
  EXP_OF : Inport  Port=3
  ERR_OUT : Outport
  wires:
  ERR_IN/1 -> ERR_OUT/1

== system untitled/Subsystem/SummingStage/RCA ==
  EXT_M1 : Inport
  SHFT_M2 : Inport  Port=2
  OP_IN : Inport  Port=3
  RESULT : Outport
  REM_MAN : Outport  Port=2
  wires:
  EXT_M1/1 -> RESULT/1

== system untitled/Subsystem/SummingStage/RCA1 ==
  PLUS_ONE : Inport
  0 : Inport  Port=2
  GRT_EXP : Inport  Port=3
  EXP_OUT : Outport
  EXP_OF : Outport  Port=2
  wires:
  PLUS_ONE/1 -> EXP_OUT/1

== system untitled/Subsystem/SummingStage/ShifterR ==
  EXT_M2 : Inport
  OFF : Inport  Port=2
  SHFT_M2 : Outport
  wires:
  EXT_M2/1 -> SHFT_M2/1

== system untitled/Subsystem/SummingStage/Subsystem1 ==
  In1 : Inport
  Out1 : Outport
  wires:
  In1/1 -> Out1/1

== system untitled/Subsystem/SummingStage/Subsystem2 ==
  RESULT : Inport
  Out1 : Outport
  wires:
  RESULT/1 -> Out1/1

== system untitled/Subsystem/SummingStage/Subsystem3 ==
  In1 : Inport
  Out1 : Outport
  wires:
  In1/1 -> Out1/1

== system untitled/Subsystem/SummingStage/Subsystem5 ==
  In1 : Inport
  Out1 : Outport
  wires:
  In1/1 -> Out1/1

== system untitled/Subsystem/AdjustingStage/Normalizer/EightBitComparator ==
  SUB_EXP : Inport
  EXP_IN : Inport  Port=2
  Constant : Constant  Value=0
  Constant1 : Constant
  Constant2 : Constant  Value=0
  FourBitComparator : Subsystem
      mask Display:
      | port_label('output', 1, 'SML_OUT');
      | port_label('output', 2, 'EQ_OUT');
      | port_label('output', 3, 'GRT_OUT');
      | port_label('input', 3, 'SML_IN');
      | port_label('input', 4, 'EQ_IN');
      | port_label('input', 5, 'GRT_IN');
  FourBitComparator1 : Subsystem
      mask Display:
      | port_label('output', 1, 'SML_OUT');
      | port_label('output', 2, 'EQ_OUT');
      | port_label('output', 3, 'GRT_OUT');
      | port_label('input', 3, 'SML_IN');
      | port_label('input', 4, 'EQ_IN');
      | port_label('input', 5, 'GRT_IN');
  Subsystem : Subsystem
      mask Display: disp('A(7 downto 4)');
  Subsystem1 : Subsystem
      mask Display: disp('B(7 downto 4)');
  Subsystem2 : Subsystem
      mask Display: disp('A(3 downto 0)');
  Subsystem3 : Subsystem
      mask Display: disp('B(3 downto 0)');
  EXP_UF : Outport
  wires:
  SUB_EXP/1 -> Subsystem1/1(In1), Subsystem3/1(In1)
  EXP_IN/1 -> Subsystem2/1(In1), Subsystem/1(In1)
  Constant1/1 -> FourBitComparator1/4(In5)
  Constant/1 -> FourBitComparator1/3(In3)
  Subsystem3/1(Out1) -> FourBitComparator1/2(In2)
  Subsystem2/1(Out1) -> FourBitComparator1/1(In1)
  FourBitComparator1/3(Out3) -> FourBitComparator/5(In4)
  Subsystem1/1(Out1) -> FourBitComparator/2(In2)
  FourBitComparator1/1(Out1) -> FourBitComparator/3(In3)
  Constant2/1 -> FourBitComparator1/5(In4)
  Subsystem/1(Out1) -> FourBitComparator/1(In1)
  FourBitComparator/1(Out1) -> EXP_UF/1
  FourBitComparator1/2(Out2) -> FourBitComparator/4(In5)

== system untitled/Subsystem/AdjustingStage/Normalizer/RCA ==
  SUB_EXP : Inport
  EXP_IN : Inport  Port=2
  In3 : Inport  Port=3
  TMP_EXP : Outport
  wires:
  EXP_IN/1 -> TMP_EXP/1

== system untitled/Subsystem/AdjustingStage/Normalizer/ReversePriorityEncoder ==
  MAN_IN : Inport
  MAN_OFF : Outport
  wires:
  MAN_IN/1 -> MAN_OFF/1

== system untitled/Subsystem/AdjustingStage/Normalizer/ShifterL ==
  MAN_IN : Inport
  MAN_OFF : Inport  Port=2
  MAN_OUT : Outport
  wires:
  MAN_IN/1 -> MAN_OUT/1

== system untitled/Subsystem/AdjustingStage/Normalizer/Subsystem ==
  In1 : Inport
  Out1 : Outport
  wires:
  In1/1 -> Out1/1

== system untitled/Subsystem/AdjustingStage/SpecialOutput/MUX ==
  In5 : Inport
  In1 : Inport  Port=2
  In2 : Inport  Port=3
  In3 : Inport  Port=4
  In4 : Inport  Port=5
  In6 : Inport  Port=6
  Out1 : Outport
  wires:
  In1/1 -> Out1/1

== system untitled/Subsystem/AdjustingStage/SpecialOutput/MUX1 ==
  In1 : Inport
  Bus Element In2 : Inport  Port=2  PortName=InBus  Element=signal1
  In3 : Inport  Port=3
  TMP_FLAG : Outport
  wires:
  In1/1 -> TMP_FLAG/1

== system untitled/Subsystem/ComparingStage/CaseManager/Subsystem ==
  In1 : Inport
  In2 : Inport  Port=2
  In3 : Inport  Port=3
  In4 : Inport  Port=4
  In5 : Inport  Port=5
  Out1 : Outport
  wires:
  In1/1 -> Out1/1

== system untitled/Subsystem/ComparingStage/CaseManager/Subsystem1 ==
  In1 : Inport
  Out1 : Outport
  wires:
  In1/1 -> Out1/1

== system untitled/Subsystem/ComparingStage/CaseManager/Subsystem2 ==
  In1 : Inport
  Out1 : Outport
  wires:
  In1/1 -> Out1/1

== system untitled/Subsystem/ComparingStage/CaseManager/Subsystem3 ==
  In1 : Inport
  Out1 : Outport
  wires:
  In1/1 -> Out1/1

== system untitled/Subsystem/ComparingStage/CaseManager/Subsystem4 ==
  In1 : Inport
  Out1 : Outport
  wires:
  In1/1 -> Out1/1

== system untitled/Subsystem/ComparingStage/CaseManager/Subsystem5 ==
  In1 : Inport
  Out1 : Outport
  wires:
  In1/1 -> Out1/1

== system untitled/Subsystem/ComparingStage/CaseManager/Subsystem6 ==
  In1 : Inport
  Out1 : Outport
  wires:
  In1/1 -> Out1/1

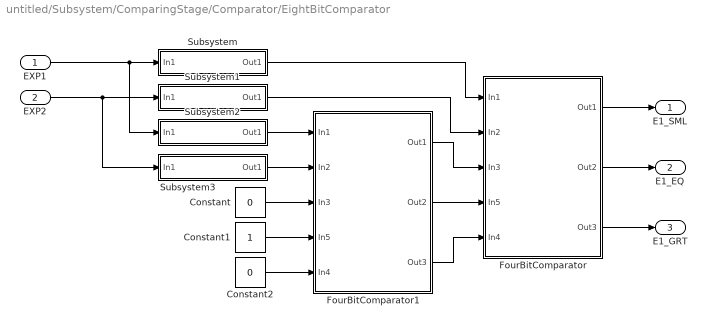
== system untitled/Subsystem/ComparingStage/Comparator/EightBitComparator ==
  EXP1 : Inport
  EXP2 : Inport  Port=2
  Constant : Constant  Value=0
  Constant1 : Constant
  Constant2 : Constant  Value=0
  FourBitComparator : Subsystem
      mask Display:
      | port_label('output', 1, 'SML_OUT');
      | port_label('output', 2, 'EQ_OUT');
      | port_label('output', 3, 'GRT_OUT');
      | port_label('input', 3, 'SML_IN');
      | port_label('input', 4, 'EQ_IN');
      | port_label('input', 5, 'GRT_IN');
  FourBitComparator1 : Subsystem
      mask Display:
      | port_label('output', 1, 'SML_OUT');
      | port_label('output', 2, 'EQ_OUT');
      | port_label('output', 3, 'GRT_OUT');
      | port_label('input', 3, 'SML_IN');
      | port_label('input', 4, 'EQ_IN');
      | port_label('input', 5, 'GRT_IN');
  Subsystem : Subsystem
      mask Display: disp('A(7 downto 4)');
  Subsystem1 : Subsystem
      mask Display: disp('B(7 downto 4)');
  Subsystem2 : Subsystem
      mask Display: disp('A(3 downto 0)');
  Subsystem3 : Subsystem
      mask Display: disp('B(3 downto 0)');
  E1_SML : Outport
  E1_EQ : Outport  Port=2
  E1_GRT : Outport  Port=3
  wires:
  FourBitComparator1/3(Out3) -> FourBitComparator/5(In4)
  Subsystem1/1(Out1) -> FourBitComparator/2(In2)
  FourBitComparator1/2(Out2) -> FourBitComparator/4(In5)
  Subsystem/1(Out1) -> FourBitComparator/1(In1)
  Constant2/1 -> FourBitComparator1/5(In4)
  FourBitComparator1/1(Out1) -> FourBitComparator/3(In3)
  Constant1/1 -> FourBitComparator1/4(In5)
  Subsystem2/1(Out1) -> FourBitComparator1/1(In1)
  Subsystem3/1(Out1) -> FourBitComparator1/2(In2)
  Constant/1 -> FourBitComparator1/3(In3)
  EXP1/1 -> Subsystem2/1(In1), Subsystem/1(In1)
  EXP2/1 -> Subsystem1/1(In1), Subsystem3/1(In1)
  FourBitComparator/1(Out1) -> E1_SML/1
  FourBitComparator/2(Out2) -> E1_EQ/1
  FourBitComparator/3(Out3) -> E1_GRT/1

== system untitled/Subsystem/ComparingStage/Comparator/MUX ==
  In1 : Inport
  In2 : Inport  Port=2
  In3 : Inport  Port=3
  Out1 : Outport
  wires:
  In1/1 -> Out1/1

== system untitled/Subsystem/ComparingStage/Comparator/MUX1 ==
  In1 : Inport
  In2 : Inport  Port=2
  In3 : Inport  Port=3
  Out1 : Outport
  wires:
  In1/1 -> Out1/1

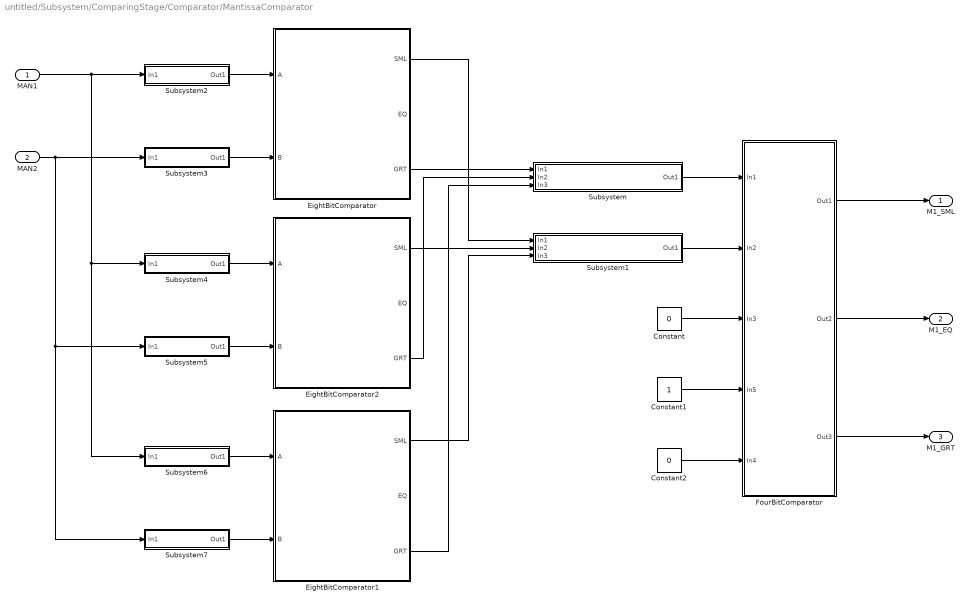
== system untitled/Subsystem/ComparingStage/Comparator/MantissaComparator ==
  MAN1 : Inport
  MAN2 : Inport  Port=2
  Constant : Constant  Value=0
  Constant1 : Constant
  Constant2 : Constant  Value=0
  EightBitComparator : Subsystem
  EightBitComparator1 : Subsystem
  EightBitComparator2 : Subsystem
  FourBitComparator : Subsystem
      mask Display:
      | port_label('output', 1, 'SML_OUT');
      | port_label('output', 2, 'EQ_OUT');
      | port_label('output', 3, 'GRT_OUT');
      | port_label('input', 3, 'SML_IN');
      | port_label('input', 4, 'EQ_IN');
      | port_label('input', 5, 'GRT_IN');
  Subsystem : Subsystem
      mask Display: disp('GRT3 & GRT2 & GRT1');
  Subsystem1 : Subsystem
      mask Display: disp('SML3 & SML2 & SML1');
  Subsystem2 : Subsystem
      mask Display: disp('A(22 downto 15)');
  Subsystem3 : Subsystem
      mask Display: disp('B(22 downto 15)');
  Subsystem4 : Subsystem
      mask Display: disp('A(14 downto 7)');
  Subsystem5 : Subsystem
      mask Display: disp('B(14 downto 7)');
  Subsystem6 : Subsystem
      mask Display: disp("A(6 downto 0) & '0'");
  Subsystem7 : Subsystem
      mask Display: disp("B(6 downto 0) & '0'");
  M1_SML : Outport
  M1_EQ : Outport  Port=2
  M1_GRT : Outport  Port=3
  wires:
  Constant/1 -> FourBitComparator/3(In3)
  Constant1/1 -> FourBitComparator/4(In5)
  Constant2/1 -> FourBitComparator/5(In4)
  FourBitComparator/1(Out1) -> M1_SML/1
  FourBitComparator/2(Out2) -> M1_EQ/1
  FourBitComparator/3(Out3) -> M1_GRT/1
  EightBitComparator/3(GRT) -> Subsystem/1(In1)
  EightBitComparator2/3(GRT) -> Subsystem/2(In2)
  EightBitComparator1/3(GRT) -> Subsystem/3(In3)
  EightBitComparator/1(SML) -> Subsystem1/1(In1)
  EightBitComparator2/1(SML) -> Subsystem1/2(In2)
  EightBitComparator1/1(SML) -> Subsystem1/3(In3)
  Subsystem/1(Out1) -> FourBitComparator/1(In1)
  Subsystem1/1(Out1) -> FourBitComparator/2(In2)
  Subsystem2/1(Out1) -> EightBitComparator/1(A)
  Subsystem3/1(Out1) -> EightBitComparator/2(B)
  Subsystem4/1(Out1) -> EightBitComparator2/1(A)
  Subsystem5/1(Out1) -> EightBitComparator2/2(B)
  Subsystem6/1(Out1) -> EightBitComparator1/1(A)
  Subsystem7/1(Out1) -> EightBitComparator1/2(B)
  MAN1/1 -> Subsystem2/1(In1), Subsystem4/1(In1), Subsystem6/1(In1)
  MAN2/1 -> Subsystem3/1(In1), Subsystem5/1(In1), Subsystem7/1(In1)

== system untitled/Subsystem/ComparingStage/Comparator/Subsystem ==
  In4 : Inport
  In5 : Inport  Port=2
  In6 : Inport  Port=3
  In1 : Inport  Port=4
  In3 : Inport  Port=5
  In2 : Inport  Port=6
  SIG_OUT_TMP : Outport
  wires:
  In1/1 -> SIG_OUT_TMP/1

== system untitled/Subsystem/ComparingStage/Comparator/Subsystem1 ==
  In1 : Inport
  Out1 : Outport
  wires:
  In1/1 -> Out1/1

== system untitled/Subsystem/ComparingStage/Comparator/Subsystem2 ==
  In1 : Inport
  Out1 : Outport
  wires:
  In1/1 -> Out1/1

== system untitled/Subsystem/ComparingStage/Comparator/Subsystem3 ==
  In1 : Inport
  Out1 : Outport
  wires:
  In1/1 -> Out1/1

== system untitled/Subsystem/ComparingStage/Comparator/Subsystem4 ==
  In1 : Inport
  Out1 : Outport
  wires:
  In1/1 -> Out1/1

== system untitled/Subsystem/ComparingStage/Comparator/Subsystem5 ==
  In1 : Inport
  Out1 : Outport
  wires:
  In1/1 -> Out1/1

== system untitled/Subsystem/ComparingStage/Comparator/Subsystem6 ==
  In1 : Inport
  Out1 : Outport
  wires:
  In1/1 -> Out1/1
